simulink model "problem3_sim"  (R2019a)
settings: Solver=VariableStepAuto  StartTime=0.0  StopTime=30  RelTol=1e-3
InitFcn:
  | w_n = 2 %rad/sec
  | zeta = 0.4 % damping ratio
  | C = [.5, 0]
values from neighbouring files (symbols this model uses):
  D_wave = 6    [problem_3.m]
  D_wind = 7    [problem_3.m]
  k = 7    [problem_1.m]    (also in problem_3.m = B'*s_inf)
  x_init = [x1_init(i), x2_init(i)]'    [problem_2.m]    (also in problem_3.m = [ 0.3, 0])
settings Model: Creator=glitch  LastModifiedBy=glitch

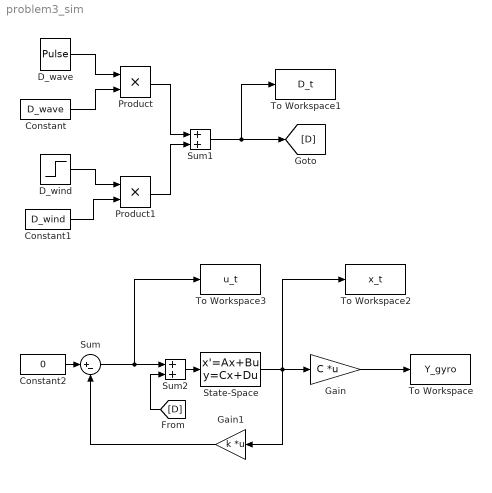
== system problem3_sim ==
  Constant : Constant  Value=D_wave
  Constant1 : Constant  Value=D_wind
  Constant2 : Constant  Value=0
  D_wave : DiscretePulseGenerator  PulseType=Time based  Period=1  PulseWidth=10
  D_wind : Step  Time=10  SampleTime=0
  Gain : Gain  Gain=C  Multiplication=Matrix(K*u)
  Gain1 : Gain  Gain=k  Multiplication=Matrix(K*u)
  Product : Product
  Product1 : Product
  State-Space : StateSpace  A=[0,1; -w_n^2, -2*w_n*zeta]  B=[0; 2*w_n^2]  C=eye(2)  D=[0;0]  InitialCondition=x_init
  Sum : Sum  Inputs=|+-
  Sum1 : Sum
  Sum2 : Sum
  To Workspace : ToWorkspace  VariableName=Y_gyro  SaveFormat=Structure With Time  SampleTime=-1
  To Workspace1 : ToWorkspace  VariableName=D_t  SaveFormat=Structure With Time  SampleTime=-1
  To Workspace2 : ToWorkspace  VariableName=x_t  SaveFormat=Structure With Time  SampleTime=-1
  To Workspace3 : ToWorkspace  VariableName=u_t  SaveFormat=Structure With Time  SampleTime=-1
  wires:
  State-Space/1 -> To Workspace2/1, Gain1/1, Gain/1
  Gain1/1 -> Sum/2
  Gain/1 -> To Workspace/1
  D_wave/1 -> Product/1
  Constant/1 -> Product/2
  D_wind/1 -> Product1/1
  Constant1/1 -> Product1/2
  Product/1 -> Sum1/1
  Product1/1 -> Sum1/2
  Sum1/1 -> [D], To Workspace1/1
  [D] -> Sum2/2
  Constant2/1 -> Sum/1
  Sum/1 -> Sum2/1, To Workspace3/1
  Sum2/1 -> State-Space/1
